simulink model "FCS"  (R2019a)
settings: Solver=VariableStepAuto  StartTime=0.0  StopTime=10.0  RelTol=1e-3
undefined symbols (not defined in the file): argentina, ground, JD_0, Jw, namibia, nut80, r_ecef, t_orbit, v_ecef
libraries: dspmathops x12, vrlib x8, sc_toolbox x7
(part 2 of 2)

== matlab function FCS/Environment/Sun Position Model /MOD to ECEF/MATLAB Function ==
  data: reci input; rteme output; ttt input; ddpsi input; ddeps input; nut80 input
% ----------------------------------------------------------------------------
%
%                           function eci2teme
%
%  this function transforms a vector from the mean equator mean equinox (j2000) 
%    system (eci), to the true equator mean equinox (teme) system.
%
%  author        : david vallado                  719-573-2600   30 oct 2017
%
%  inputs          description                    range / units
%    reci        - position vector eci            km
%    veci        - velocity vector eci            km/s
%    aeci        - acceleration vector eci        km/s2
%    ttt         - julian centuries of tt         centuries
%    ddpsi       - delta psi correction to gcrf   rad
%    ddeps       - delta eps correction to gcrf   rad
%
%  outputs       :
%    rteme       - position vector of date
%                    true equator, mean equinox   km
%    vteme       - velocity vector of date
%                    true equator, mean equinox   km/s
%    ateme       - acceleration vector of date
%                    true equator, mean equinox   km/s2
%
%  locals        :
%    prec        - matrix for eci - mod
%    nutteme     - matrix for mod - teme - an approximation for nutation
%    eqe         - rotation for equation of equinoxes (geometric terms only)
%    tm          - combined matrix for teme2eci
%
%  coupling      :
%   precess      - rotation for precession        eci - mod
%   nutation     - rotation for nutation          eci - tod
%
%  references    :
%    vallado       2013, 231-233
%
% [reci, veci, aeci] = teme2eci  ( rteme, vteme, ateme, ttt, ddpsi, ddeps);
% ----------------------------------------------------------------------------

function rteme  = eci2teme  ( reci, ttt, ddpsi, ddeps, nut80)

        [prec,psia, wa, ea, xa] = precess ( ttt);

        [deltapsi, trueeps, meaneps, omega, nut] = nutation  (ttt, ddpsi, ddeps, nut80 );
        
        % ------------------------ find eqeg ----------------------
        % rotate teme through just geometric terms 
        eqeg = deltapsi* cos(meaneps);

        eqeg = rem (eqeg, 2.0*pi);
        eqe = zeros(3,3);
        eqe(1,1) =  cos(eqeg);
        eqe(1,2) =  sin(eqeg);
        eqe(1,3) =  0.0;
        eqe(2,1) = -sin(eqeg);
        eqe(2,2) =  cos(eqeg);
        eqe(2,3) =  0.0;
        eqe(3,1) =  0.0;
        eqe(3,2) =  0.0;
        eqe(3,3) =  1.0;

        tm = eqe * nut' * prec';
        
        rteme = tm * reci;
 
        


%�
% ----------------------------------------------------------------------------
%
%                           function precess
%
%  this function calulates the transformation matrix that accounts for the effects
%    of precession. both the 1980 and 2000 theories are handled. note that the 
%    required parameters differ a little. 
%
%  author        : david vallado                  719-573-2600   25 jun 2002
%
%  revisions
%    vallado     - consolidate with iau 2000                     14 feb 2005
%
%  inputs          description                    range / units
%    ttt         - julian centuries of tt
%    opt         - method option                  '01', '02', '96', '80'
%
%  outputs       :
%    prec        - transformation matrix for mod - j2000 (80 only)
%    psia        - cannonical precession angle    rad    (00 only)
%    wa          - cannonical precession angle    rad    (00 only)
%    ea          - cannonical precession angle    rad    (00 only)
%    xa          - cannonical precession angle    rad    (00 only)
%
%  locals        :
%    ttt2        - ttt squared
%    ttt3        - ttt cubed
%    zeta        - precession angle               rad
%    z           - precession angle               rad
%    theta       - precession angle               rad
%    oblo        - obliquity value at j2000 epoch "%
%
%  coupling      :
%    none        -
%
%  references    :
%    vallado       2004, 214-216, 219-221
%
% [prec,psia,wa,ea,xa] = precess ( ttt, opt );
% ----------------------------------------------------------------------------

function [prec,psia,wa,ea,xa] = precess ( ttt );

       % sethelp;
        
        % " to rad
        convrt = pi / (180.0*3600.0);
        ttt2= ttt * ttt;
        ttt3= ttt2 * ttt;

        % ------------------- fk4 b1950 precession angles --------------------
%         if (opt == '50')
% 
%             % ---- Seidelmann pg 107             
%             % for these calls, ttt will come in with the current jd
% %            t1= 0.0; %(ttt - 2433282.42345905)/365242.198782;  % set start as B1850, 0.0 to simplify
% %            t2= (ttt - 2396758.203)/365242.198782;  % uses B1850
% %            ttt = t2 - t1;
% %            ttt2 = ttt * ttt;
% %            ttt3 = ttt * ttt2;
% %            fprintf(1,'50prec %15.9f  \n',ttt);
%             % exp supp 61 pg 38
% %            psia = 50.3708 + 0.0050 * ttt;
% %            wa = 0.0;
% %            ea = 0.0;
% %            xa = 0.1247 - 0.0188 * ttt;
% %            zeta =  (23035.545 + 139.720*t1 + 0.060 *t1*t1)*ttt + (30.240-0.270*t1)*ttt2 + 17.995*ttt3; % "
% %            theta=  (20051.12 - 85.29*t1 - 0.37 *t1*t1)*ttt + (-42.65-0.37*t1)*ttt2 - 41.80*ttt3;
% %            z    =  (23035.545 + 139.720*t1 + 0.060 *t1*t1)*ttt + (109.480+0.390*t1)*ttt2 + 18.325*ttt3;
% 
%             % ---- Newcomb Exp Supp 61 approach, but see GTDS pg 3-17
%             % Exp Supp 61 says use 1900? but gtds says use 1950. 
%             % for these calls, ttt will come in with the current jd
%             t1= 0.0; %(ttt - 2415020.31352)/36524.2198782;  % set start as B1900, 0.0 to simplify
% %            t2= (ttt - 2415020.31352)/36525;  % uses B1900   
%             t2= (ttt - 2433282.42345905)/36525;  % uses B1950  
% %            ttt = t2 - t1;
% %            ttt2 = ttt * ttt;
% %            ttt3 = ttt * ttt2;
%             % exp supp 61 pg 38
%             psia = 50.3708 + 0.0050 * ttt;
%             wa = 0.0; % not sure which one is which...
%             ea = 84428.26 -   46.845*ttt - 0.00059*ttt2 + 0.00181*ttt3;
%             xa = 0.1247 - 0.0188 * ttt;
%            fprintf(1,'50prec %15.9f  \n',ttt);
%            % seems like Exp supp 61 is ok with 1900 as epoch, and Seidlemann is ok with listed measr,  
% %            zeta =  (2304.25 + 1.396*t1)*ttt + 0.302*ttt2 + 0.018*ttt3; % "
% %            theta=  (2004.682 - 0.853*t1)*ttt -0.426*ttt2 - 0.042*ttt3;
% %            z    =  (2304.25 + 1.396*t1)*ttt + 1.093*ttt2 + 0.018*ttt3;
%             % GTDS pg 3-17 using days from 1950 - avoids long rpecession
%             % constants...
%             zeta =  2304.9969*ttt + 0.302*ttt2 + 0.01808*ttt3; % "
%             theta=  2004.2980*ttt -0.425936*ttt2 - 0.0416*ttt3;
%             z    =  2304.9969*ttt + 1.092999*ttt2 + 0.0192*ttt3;
%             
% 
%             % tp-008 36-45
%             % ttt is tropical centruies from 1950 36524.22 days
%             prec = zeros(3,3);
%             prec(1,1) =  1.0 - 2.9696e-4 * ttt2 - 1.3e-7 * ttt3;
%             prec(1,2) =  2.234941e-2 * ttt + 6.76e-6 * ttt2 - 2.21e-6 * ttt3;
%             prec(1,3) =  9.7169e-3 * ttt - 2.07e-6 * ttt2 - 9.6e-7 * ttt3;
%             prec(2,1) =  -prec(1,2);
%             prec(2,2) =  1.0 - 2.4975e-4 * ttt2 - 1.5e-7 * ttt3;
%             prec(2,3) =  - 1.0858e-4 * ttt2;
%             prec(3,1) =  -prec(1,3);
%             prec(3,2) =  prec(2,3);
%             prec(3,3) =  1.0 - 4.721e-5 * ttt2;
%  
%             
%            % pass these back out for testing
%            psia = zeta;
%            wa = theta;
%            ea = z;
%         % ------------------- iau 76 precession angles --------------------
%         else
%           if (opt == '80')
%     fprintf(1,'80prec %15.9f  \n',ttt);
            psia =             5038.7784*ttt - 1.07259*ttt2 - 0.001147*ttt3; % "
            wa   = 84381.448                 + 0.05127*ttt2 - 0.007726*ttt3;
            ea   = 84381.448 -   46.8150*ttt - 0.00059*ttt2 + 0.001813*ttt3;
            xa   =               10.5526*ttt - 2.38064*ttt2 - 0.001125*ttt3;
            zeta =             2306.2181*ttt + 0.30188*ttt2 + 0.017998*ttt3; % "
            theta=             2004.3109*ttt - 0.42665*ttt2 - 0.041833*ttt3;
            z    =             2306.2181*ttt + 1.09468*ttt2 + 0.018203*ttt3;
          % ------------------ iau 03 precession angles -------------------
%           else
%             oblo =  84381.406; % "
%             psia =  (((( -0.0000000951 * ttt + 0.000132851 ) * ttt - 0.00114045 ) * ttt - 1.0790069 ) * ttt + 5038.481507 ) * ttt; % "
%             wa   =  ((((  0.0000003337 * ttt - 0.000000467 ) * ttt - 0.00772503 ) * ttt + 0.0512623 ) * ttt -    0.025754 ) * ttt + oblo;
%             ea   =  (((( -0.0000000434 * ttt - 0.000000576 ) * ttt + 0.00200340 ) * ttt - 0.0001831 ) * ttt -   46.836769 ) * ttt + oblo;
%             xa   =  (((( - 0.0000000560 * ttt + 0.000170663 ) * ttt - 0.00121197 ) * ttt - 2.3814292 ) * ttt +   10.556403 ) * ttt;
% 
%             zeta =  (((( - 0.0000003173 * ttt - 0.000005971 ) * ttt + 0.01801828 ) * ttt + 0.2988499 ) * ttt + 2306.083227 ) * ttt + 2.650545; % "
%             theta=  (((( - 0.0000001274 * ttt - 0.000007089 ) * ttt - 0.04182264 ) * ttt - 0.4294934 ) * ttt + 2004.191903 ) * ttt;
%             z    =  ((((   0.0000002904 * ttt - 0.000028596 ) * ttt + 0.01826837 ) * ttt + 1.0927348 ) * ttt + 2306.077181 ) * ttt - 2.650545;
%           end;
%         end;
        
        % convert units to rad
        psia = psia  * convrt; % rad
        wa   = wa    * convrt;
        ea   = ea    * convrt;
        xa   = xa    * convrt;
        zeta = zeta  * convrt; 
        theta= theta * convrt;
        z    = z     * convrt;
%iauhelp='y';         
%fprintf(1,'pr %11.7f  %11.7f  %11.7fdeg \n',zeta*180/pi,theta*180/pi,z*180/pi );
%         if (iauhelp == 'y')
%             fprintf(1,'pr %11.7f  %11.7f  %11.7f %11.7fdeg \n',psia*180/pi,wa*180/pi,ea*180/pi,xa*180/pi );
%             fprintf(1,'pr %11.7f  %11.7f  %11.7fdeg \n',zeta*180/pi,theta*180/pi,z*180/pi );
%         end;
% 
%         if (strcmp(opt,'80')==1) % || (strcmp(opt,'50') == 1)
            coszeta  = cos(zeta);
            sinzeta  = sin(zeta);
            costheta = cos(theta);
            sintheta = sin(theta);
            cosz     = cos(z);
            sinz     = sin(z);

            % ----------------- form matrix  mod to j2000 -----------------
            prec = zeros(3,3);
            prec(1,1) =  coszeta * costheta * cosz - sinzeta * sinz;
            prec(1,2) =  coszeta * costheta * sinz + sinzeta * cosz;
            prec(1,3) =  coszeta * sintheta;
            prec(2,1) = -sinzeta * costheta * cosz - coszeta * sinz;
            prec(2,2) = -sinzeta * costheta * sinz + coszeta * cosz;
            prec(2,3) = -sinzeta * sintheta;
            prec(3,1) = -sintheta * cosz;
            prec(3,2) = -sintheta * sinz;
            prec(3,3) =  costheta;

            % ----------------- do rotations instead ----------------------
            % p1 = rot3mat( z );
            % p2 = rot2mat( -theta );
            % p3 = rot3mat( zeta );
            % prec = p3*p2*p1;
%         elseif (strcmp(opt,'50') ~= 1)
%             oblo = oblo * convrt; % " to rad
%             a4  = rot3mat(-xa);
%             a5  = rot1mat(wa);
%             a6  = rot3mat(psia);
%             a7  = rot1mat(-oblo);
%             prec = a7*a6*a5*a4;
%            % prec = zeros(3);
%         end;



% ----------------------------------------------------------------------------
%
%                           function nutation
%
%  this function calulates the transformation matrix that accounts for the
%    effects of nutation.
%
%  author        : david vallado                  719-573-2600   27 jun 2002
%
%  revisions
%    vallado     - consolidate with iau 2000                     14 feb 2005
%
%  inputs          description                    range / units
%    ttt         - julian centuries of tt
%    ddpsi       - delta psi correction to gcrf   rad
%    ddeps       - delta eps correction to gcrf   rad
%
%  outputs       :
%    deltapsi    - nutation angle                 rad
%    trueeps     - true obliquity of the ecliptic rad
%    meaneps     - mean obliquity of the ecliptic rad
%    omega       -                                rad
%    nut         - transformation matrix for tod - mod
%
%  locals        :
%    iar80       - integers for fk5 1980
%    rar80       - reals for fk5 1980
%    ttt2        - ttt squared
%    ttt3        - ttt cubed
%    l           -                                rad
%    ll          -                                rad
%    f           -                                rad
%    d           -                                rad
%    deltaeps    - change in obliquity            rad
%
%  coupling      :
%    fundarg     - find fundamental arguments
%
%  references    :
%    vallado       2013, 224-226
%
% [deltapsi, trueeps, meaneps, omega,nut] = nutation  (ttt, ddpsi, ddeps );
% ----------------------------------------------------------------------------

function [deltapsi, trueeps, meaneps, omega,nut] = nutation  (ttt, ddpsi, ddeps , nut80);

        deg2rad = pi/180.0;

        [iar80,rar80] =  iau80in(nut80);  % coeff in deg

        % ---- determine coefficients for iau 1980 nutation theory ----
        ttt2= ttt*ttt;
        ttt3= ttt2*ttt;

        meaneps = -46.8150 *ttt - 0.00059 *ttt2 + 0.001813 *ttt3 + 84381.448;
        meaneps = rem( meaneps/3600.0, 360.0 );
        meaneps = meaneps * deg2rad;

        [ l, l1, f, d, omega, ...
          lonmer, lonven, lonear, lonmar, lonjup, lonsat, lonurn, lonnep, precrate ...
        ] = fundarg( ttt, '80' );
%fprintf(1,'nut del arg %11.7f  %11.7f  %11.7f  %11.7f  %11.7f  \n',l*180/pi,l1*180/pi,f*180/pi,d*180/pi,omega*180/pi );

        deltapsi= 0.0;
        deltaeps= 0.0;
        for i= 106:-1: 1
            tempval= iar80(i,1)*l + iar80(i,2)*l1 + iar80(i,3)*f + ...
                     iar80(i,4)*d + iar80(i,5)*omega;
            deltapsi= deltapsi + (rar80(i,1)+rar80(i,2)*ttt) * sin( tempval );
            deltaeps= deltaeps + (rar80(i,3)+rar80(i,4)*ttt) * cos( tempval );
        end

        % --------------- find nutation parameters --------------------
        deltapsi = rem( deltapsi + ddpsi, 2.0 * pi );
        deltaeps = rem( deltaeps + ddeps, 2.0 * pi );
        trueeps  = meaneps + deltaeps;

%fprintf(1,'meaneps %11.7f dp  %11.7f de  %11.7f te  %11.7f  ttt  %11.7f \n',meaneps*180/pi,deltapsi*180/pi,deltaeps*180/pi,trueeps*180/pi, ttt );

        cospsi  = cos(deltapsi);
        sinpsi  = sin(deltapsi);
        coseps  = cos(meaneps);
        sineps  = sin(meaneps);
        costrueeps = cos(trueeps);
        sintrueeps = sin(trueeps);
        
        nut = zeros(3,3);
        nut(1,1) =  cospsi;
        nut(1,2) =  costrueeps * sinpsi;
        nut(1,3) =  sintrueeps * sinpsi;
        nut(2,1) = -coseps * sinpsi;
        nut(2,2) =  costrueeps * coseps * cospsi + sintrueeps * sineps;
        nut(2,3) =  sintrueeps * coseps * cospsi - sineps * costrueeps;
        nut(3,1) = -sineps * sinpsi;
        nut(3,2) =  costrueeps * sineps * cospsi - sintrueeps * coseps;
        nut(3,3) =  sintrueeps * sineps * cospsi + costrueeps * coseps;

      %   n1 = rot1mat( trueeps );
      %   n2 = rot3mat( deltapsi );
      %   n3 = rot1mat( -meaneps );
      %   nut = n3*n2*n1

%�
% ----------------------------------------------------------------------------
%
%                           function fundarg
%
%  this function calulates the delauany variables and planetary values for
%  several theories.
%
%  author        : david vallado                  719-573-2600   16 jul 2004
%
%  revisions
%    vallado     - consolidate with iau 2000                     14 feb 2005
%
%  inputs          description                    range / units
%    ttt         - julian centuries of tt
%    opt         - method option                  '10', '02', '96', '80'
%
%  outputs       :
%    l           - delaunay element               rad
%    ll          - delaunay element               rad
%    f           - delaunay element               rad
%    d           - delaunay element               rad
%    omega       - delaunay element               rad
%    planetary longitudes                         rad
%
%  locals        :
%    ttt2,ttt3,  - powers of ttt
%
%  coupling      :
%    none        -
%
%  references    :
%    vallado       2004, 212-214
%
% [ l, l1, f, d, omega, ...
%   lonmer, lonven, lonear, lonmar, lonjup, lonsat, lonurn, lonnep, precrate ...
% ] = fundarg( ttt, opt );
% ----------------------------------------------------------------------------

function [ l, l1, f, d, omega, ...
           lonmer, lonven, lonear, lonmar, lonjup, lonsat, lonurn, lonnep, precrate ...
         ] = fundarg( ttt, opt )

        %sethelp;

        deg2rad = pi/180.0;

        % ---- determine coefficients for iau 2000 nutation theory ----
        ttt2 = ttt*ttt;
        ttt3 = ttt2*ttt;
        ttt4 = ttt2*ttt2;

        % ---- iau 2010 theory
        if opt == '10'
            % ------ form the delaunay fundamental arguments in deg
            l    =  134.96340251  + ( 1717915923.2178 *ttt + ...
                     31.8792 *ttt2 + 0.051635 *ttt3 - 0.00024470 *ttt4 ) / 3600.0;
            l1   =  357.52910918  + (  129596581.0481 *ttt - ...
                      0.5532 *ttt2 - 0.000136 *ttt3 - 0.00001149*ttt4 )  / 3600.0;
            f    =   93.27209062  + ( 1739527262.8478 *ttt - ...
                     12.7512 *ttt2 + 0.001037 *ttt3 + 0.00000417*ttt4 )  / 3600.0;
            d    =  297.85019547  + ( 1602961601.2090 *ttt - ...
                      6.3706 *ttt2 + 0.006593 *ttt3 - 0.00003169*ttt4 )  / 3600.0;
            omega=  125.04455501  + (   -6962890.5431 *ttt + ...
                      7.4722 *ttt2 + 0.007702 *ttt3 - 0.00005939*ttt4 )  / 3600.0;

            % ------ form the planetary arguments in deg
            lonmer  = 252.250905494  + 149472.6746358  *ttt;
            lonven  = 181.979800853  +  58517.8156748  *ttt;
            lonear  = 100.466448494  +  35999.3728521  *ttt;
            lonmar  = 355.433274605  +  19140.299314   *ttt;
            lonjup  =  34.351483900  +   3034.90567464 *ttt;
            lonsat  =  50.0774713998 +   1222.11379404 *ttt;
            lonurn  = 314.055005137  +    428.466998313*ttt;
            lonnep  = 304.348665499  +    218.486200208*ttt;
            precrate=   1.39697137214*ttt + 0.0003086*ttt2;
         end;

        % ---- iau 2000b theory
        if opt == '02'
            % ------ form the delaunay fundamental arguments in deg
            l    =  134.96340251  + ( 1717915923.2178 *ttt ) / 3600.0;
            l1   =  357.52910918  + (  129596581.0481 *ttt ) / 3600.0;
            f    =   93.27209062  + ( 1739527262.8478 *ttt ) / 3600.0;
            d    =  297.85019547  + ( 1602961601.2090 *ttt ) / 3600.0;
            omega=  125.04455501  + (   -6962890.5431 *ttt ) / 3600.0;

            % ------ form the planetary arguments in deg
            lonmer  = 0.0;
            lonven  = 0.0;
            lonear  = 0.0;
            lonmar  = 0.0;
            lonjup  = 0.0;
            lonsat  = 0.0;
            lonurn  = 0.0;
            lonnep  = 0.0;
            precrate= 0.0;
         end;   

        % ---- iau 1996 theory
        if opt == '96'
            l    =  134.96340251  + ( 1717915923.2178 *ttt + ...
                     31.8792 *ttt2 + 0.051635 *ttt3 - 0.00024470 *ttt4 ) / 3600.0;
            l1   =  357.52910918  + (  129596581.0481 *ttt - ...
                      0.5532 *ttt2 - 0.000136 *ttt3 - 0.00001149*ttt4 )  / 3600.0;
            f    =   93.27209062  + ( 1739527262.8478 *ttt - ...
                     12.7512 *ttt2 + 0.001037 *ttt3 + 0.00000417*ttt4 )  / 3600.0;
            d    =  297.85019547  + ( 1602961601.2090 *ttt - ...
                      6.3706 *ttt2 + 0.006593 *ttt3 - 0.00003169*ttt4 )  / 3600.0;
            omega=  125.04455501  + (   -6962890.2665 *ttt + ...
                      7.4722 *ttt2 + 0.007702 *ttt3 - 0.00005939*ttt4 )  / 3600.0;
            % ------ form the planetary arguments in deg
            lonmer  = 0.0;
            lonven  = 181.979800853  +  58517.8156748  *ttt;   % deg
            lonear  = 100.466448494  +  35999.3728521  *ttt;
            lonmar  = 355.433274605  +  19140.299314   *ttt;
            lonjup  =  34.351483900  +   3034.90567464 *ttt;
            lonsat  =  50.0774713998 +   1222.11379404 *ttt;
            lonurn  = 0.0;
            lonnep  = 0.0;
            precrate=   1.39697137214*ttt + 0.0003086*ttt2;
         end;   

         % ---- iau 1980 theory
        if opt == '80'
            l = ((((0.064) * ttt + 31.310) * ttt + 1717915922.6330) * ttt) / 3600.0 + 134.96298139;
    		l1 = ((((-0.012) * ttt - 0.577) * ttt + 129596581.2240) * ttt) / 3600.0 + 357.52772333;
    		f = ((((0.011) * ttt - 13.257) * ttt + 1739527263.1370) * ttt) / 3600.0 + 93.27191028;
	    	d = ((((0.019) * ttt - 6.891) * ttt + 1602961601.3280) * ttt) / 3600.0 + 297.85036306;
    		omega = ((((0.008) * ttt + 7.455) * ttt - 6962890.5390) * ttt) / 3600.0 + 125.04452222;
                  
            % ------ form the planetary arguments in deg
            lonmer  = 252.3 + 149472.0 *ttt;
            lonven  = 179.9 +  58517.8 *ttt;   % deg
            lonear  =  98.4 +  35999.4 *ttt;
            lonmar  = 353.3 +  19140.3 *ttt;
            lonjup  =  32.3 +   3034.9 *ttt;
            lonsat  =  48.0 +   1222.1 *ttt;
            lonurn  =   0.0;
            lonnep  =   0.0;
            precrate=   0.0;
         end;   

        % ---- convert units to rad
        l    = rem( l,360.0  )     * deg2rad; % rad
        l1   = rem( l1,360.0  )    * deg2rad;
        f    = rem( f,360.0  )     * deg2rad;
        d    = rem( d,360.0  )     * deg2rad;
        omega= rem( omega,360.0  ) * deg2rad;

        lonmer= rem( lonmer,360.0 ) * deg2rad;  % rad
        lonven= rem( lonven,360.0 ) * deg2rad;
        lonear= rem( lonear,360.0 ) * deg2rad;
        lonmar= rem( lonmar,360.0 ) * deg2rad;
        lonjup= rem( lonjup,360.0 ) * deg2rad;
        lonsat= rem( lonsat,360.0 ) * deg2rad;
        lonurn= rem( lonurn,360.0 ) * deg2rad;
        lonnep= rem( lonnep,360.0 ) * deg2rad;
        precrate= rem( precrate,360.0 ) * deg2rad;
%iauhelp='y';
%         if iauhelp == 'y'
%             fprintf(1,'fa %11.7f  %11.7f  %11.7f  %11.7f  %11.7f deg \n',l*180/pi,l1*180/pi,f*180/pi,d*180/pi,omega*180/pi );
%             fprintf(1,'fa %11.7f  %11.7f  %11.7f  %11.7f deg \n',lonmer*180/pi,lonven*180/pi,lonear*180/pi,lonmar*180/pi );
%             fprintf(1,'fa %11.7f  %11.7f  %11.7f  %11.7f deg \n',lonjup*180/pi,lonsat*180/pi,lonurn*180/pi,lonnep*180/pi );
%             fprintf(1,'fa %11.7f  \n',precrate*180/pi );
%           end;

function [iar80,rar80] = iau80in(nut80);

       % ------------------------  implementation   -------------------
       % 0.0001" to rad
       convrt= 0.0001 * pi / (180*3600.0);

       %load nut80.dat;

       iar80 = nut80(:,1:5);
       rar80 = nut80(:,6:9);

       for i=1:106
           for j=1:4
               rar80(i,j)= rar80(i,j) * convrt;
           end
       end

== matlab function FCS/Environment/Sun Position Model /MOD to ECEF/MOD to ECI ==
  data: rmod input; reci output; ttt input
% ----------------------------------------------------------------------------
%
%                           function mod2eci
%
%  this function transforms a vector from the mean equator mean equinox of
%    date (mod) to the mean equator mean equinox (j2000) frame.
%
%  author        : david vallado                  719-573-2600   25 jun 2002
%
%  revisions
%    vallado     - consolidate with iau 2000                     14 feb 2005
%
%  inputs          description                    range / units
%    rmod        - position vector of date
%                    mean equator, mean equinox   km
%    vmod        - velocity vector of date
%                    mean equator, mean equinox   km/s
%    amod        - acceleration vector of date
%                    mean equator, mean equinox   km/s2
%    ttt         - julian centuries of tt         centuries
%
%  outputs       :
%    reci        - position vector eci            km
%    veci        - velocity vector eci            km/s
%    aeci        - acceleration vector eci        km/s2
%
%  locals        :
%    none.
%
%  coupling      :
%   precess      - rotation for precession        mod - eci
%
%  references    :
%    vallado       2001, 219-220, eq 3-68
%
% [reci,veci,aeci] = mod2eci  ( rmod,vmod,amod,ttt );
% ----------------------------------------------------------------------------

function reci  = mod2eci  ( rmod,ttt )
        
        
        [prec,psia,wa,ea,xa] = precess1 ( ttt);

        reci = prec*rmod;
        
        
        
        
        % ----------------------------------------------------------------------------
%
%                           function precess
%
%  this function calulates the transformation matrix that accounts for the effects
%    of precession. both the 1980 and 2000 theories are handled. note that the 
%    required parameters differ a little. 
%
%  author        : david vallado                  719-573-2600   25 jun 2002
%
%  revisions
%    vallado     - consolidate with iau 2000                     14 feb 2005
%
%  inputs          description                    range / units
%    ttt         - julian centuries of tt
%    opt         - method option                  '01', '02', '96', '80'
%
%  outputs       :
%    prec        - transformation matrix for mod - j2000 (80 only)
%    psia        - cannonical precession angle    rad    (00 only)
%    wa          - cannonical precession angle    rad    (00 only)
%    ea          - cannonical precession angle    rad    (00 only)
%    xa          - cannonical precession angle    rad    (00 only)
%
%  locals        :
%    ttt2        - ttt squared
%    ttt3        - ttt cubed
%    zeta        - precession angle               rad
%    z           - precession angle               rad
%    theta       - precession angle               rad
%    oblo        - obliquity value at j2000 epoch "%
%
%  coupling      :
%    none        -
%
%  references    :
%    vallado       2004, 214-216, 219-221
%
% [prec,psia,wa,ea,xa] = precess ( ttt, opt );
% ----------------------------------------------------------------------------

function [prec,psia,wa,ea,xa] = precess1 ( ttt );

       % sethelp;
        
        % " to rad
        convrt = pi / (180.0*3600.0);
        ttt2= ttt * ttt;
        ttt3= ttt2 * ttt;

        % ------------------- fk4 b1950 precession angles --------------------
%         if (opt == '50')
% 
%             % ---- Seidelmann pg 107             
%             % for these calls, ttt will come in with the current jd
% %            t1= 0.0; %(ttt - 2433282.42345905)/365242.198782;  % set start as B1850, 0.0 to simplify
% %            t2= (ttt - 2396758.203)/365242.198782;  % uses B1850
% %            ttt = t2 - t1;
% %            ttt2 = ttt * ttt;
% %            ttt3 = ttt * ttt2;
% %            fprintf(1,'50prec %15.9f  \n',ttt);
%             % exp supp 61 pg 38
% %            psia = 50.3708 + 0.0050 * ttt;
% %            wa = 0.0;
% %            ea = 0.0;
% %            xa = 0.1247 - 0.0188 * ttt;
% %            zeta =  (23035.545 + 139.720*t1 + 0.060 *t1*t1)*ttt + (30.240-0.270*t1)*ttt2 + 17.995*ttt3; % "
% %            theta=  (20051.12 - 85.29*t1 - 0.37 *t1*t1)*ttt + (-42.65-0.37*t1)*ttt2 - 41.80*ttt3;
% %            z    =  (23035.545 + 139.720*t1 + 0.060 *t1*t1)*ttt + (109.480+0.390*t1)*ttt2 + 18.325*ttt3;
% 
%             % ---- Newcomb Exp Supp 61 approach, but see GTDS pg 3-17
%             % Exp Supp 61 says use 1900? but gtds says use 1950. 
%             % for these calls, ttt will come in with the current jd
%             t1= 0.0; %(ttt - 2415020.31352)/36524.2198782;  % set start as B1900, 0.0 to simplify
% %            t2= (ttt - 2415020.31352)/36525;  % uses B1900   
%             t2= (ttt - 2433282.42345905)/36525;  % uses B1950  
% %            ttt = t2 - t1;
% %            ttt2 = ttt * ttt;
% %            ttt3 = ttt * ttt2;
%             % exp supp 61 pg 38
%             psia = 50.3708 + 0.0050 * ttt;
%             wa = 0.0; % not sure which one is which...
%             ea = 84428.26 -   46.845*ttt - 0.00059*ttt2 + 0.00181*ttt3;
%             xa = 0.1247 - 0.0188 * ttt;
%            fprintf(1,'50prec %15.9f  \n',ttt);
%            % seems like Exp supp 61 is ok with 1900 as epoch, and Seidlemann is ok with listed measr,  
% %            zeta =  (2304.25 + 1.396*t1)*ttt + 0.302*ttt2 + 0.018*ttt3; % "
% %            theta=  (2004.682 - 0.853*t1)*ttt -0.426*ttt2 - 0.042*ttt3;
% %            z    =  (2304.25 + 1.396*t1)*ttt + 1.093*ttt2 + 0.018*ttt3;
%             % GTDS pg 3-17 using days from 1950 - avoids long rpecession
%             % constants...
%             zeta =  2304.9969*ttt + 0.302*ttt2 + 0.01808*ttt3; % "
%             theta=  2004.2980*ttt -0.425936*ttt2 - 0.0416*ttt3;
%             z    =  2304.9969*ttt + 1.092999*ttt2 + 0.0192*ttt3;
%             
% 
%             % tp-008 36-45
%             % ttt is tropical centruies from 1950 36524.22 days
%             prec = zeros(3,3);
%             prec(1,1) =  1.0 - 2.9696e-4 * ttt2 - 1.3e-7 * ttt3;
%             prec(1,2) =  2.234941e-2 * ttt + 6.76e-6 * ttt2 - 2.21e-6 * ttt3;
%             prec(1,3) =  9.7169e-3 * ttt - 2.07e-6 * ttt2 - 9.6e-7 * ttt3;
%             prec(2,1) =  -prec(1,2);
%             prec(2,2) =  1.0 - 2.4975e-4 * ttt2 - 1.5e-7 * ttt3;
%             prec(2,3) =  - 1.0858e-4 * ttt2;
%             prec(3,1) =  -prec(1,3);
%             prec(3,2) =  prec(2,3);
%             prec(3,3) =  1.0 - 4.721e-5 * ttt2;
%  
%             
%            % pass these back out for testing
%            psia = zeta;
%            wa = theta;
%            ea = z;
%         % ------------------- iau 76 precession angles --------------------
%         else
%           if (opt == '80')
%     fprintf(1,'80prec %15.9f  \n',ttt);
            psia =             5038.7784*ttt - 1.07259*ttt2 - 0.001147*ttt3; % "
            wa   = 84381.448                 + 0.05127*ttt2 - 0.007726*ttt3;
            ea   = 84381.448 -   46.8150*ttt - 0.00059*ttt2 + 0.001813*ttt3;
            xa   =               10.5526*ttt - 2.38064*ttt2 - 0.001125*ttt3;
            zeta =             2306.2181*ttt + 0.30188*ttt2 + 0.017998*ttt3; % "
            theta=             2004.3109*ttt - 0.42665*ttt2 - 0.041833*ttt3;
            z    =             2306.2181*ttt + 1.09468*ttt2 + 0.018203*ttt3;
          % ------------------ iau 03 precession angles -------------------
%           else
%             oblo =  84381.406; % "
%             psia =  (((( -0.0000000951 * ttt + 0.000132851 ) * ttt - 0.00114045 ) * ttt - 1.0790069 ) * ttt + 5038.481507 ) * ttt; % "
%             wa   =  ((((  0.0000003337 * ttt - 0.000000467 ) * ttt - 0.00772503 ) * ttt + 0.0512623 ) * ttt -    0.025754 ) * ttt + oblo;
%             ea   =  (((( -0.0000000434 * ttt - 0.000000576 ) * ttt + 0.00200340 ) * ttt - 0.0001831 ) * ttt -   46.836769 ) * ttt + oblo;
%             xa   =  (((( - 0.0000000560 * ttt + 0.000170663 ) * ttt - 0.00121197 ) * ttt - 2.3814292 ) * ttt +   10.556403 ) * ttt;
% 
%             zeta =  (((( - 0.0000003173 * ttt - 0.000005971 ) * ttt + 0.01801828 ) * ttt + 0.2988499 ) * ttt + 2306.083227 ) * ttt + 2.650545; % "
%             theta=  (((( - 0.0000001274 * ttt - 0.000007089 ) * ttt - 0.04182264 ) * ttt - 0.4294934 ) * ttt + 2004.191903 ) * ttt;
%             z    =  ((((   0.0000002904 * ttt - 0.000028596 ) * ttt + 0.01826837 ) * ttt + 1.0927348 ) * ttt + 2306.077181 ) * ttt - 2.650545;
%           end;
%         end;
        
        % convert units to rad
        psia = psia  * convrt; % rad
        wa   = wa    * convrt;
        ea   = ea    * convrt;
        xa   = xa    * convrt;
        zeta = zeta  * convrt; 
        theta= theta * convrt;
        z    = z     * convrt;
%iauhelp='y';         
%fprintf(1,'pr %11.7f  %11.7f  %11.7fdeg \n',zeta*180/pi,theta*180/pi,z*180/pi );
%         if (iauhelp == 'y')
%             fprintf(1,'pr %11.7f  %11.7f  %11.7f %11.7fdeg \n',psia*180/pi,wa*180/pi,ea*180/pi,xa*180/pi );
%             fprintf(1,'pr %11.7f  %11.7f  %11.7fdeg \n',zeta*180/pi,theta*180/pi,z*180/pi );
%         end;
% 
%         if (strcmp(opt,'80')==1) % || (strcmp(opt,'50') == 1)
            coszeta  = cos(zeta);
            sinzeta  = sin(zeta);
            costheta = cos(theta);
            sintheta = sin(theta);
            cosz     = cos(z);
            sinz     = sin(z);

            % ----------------- form matrix  mod to j2000 -----------------
            prec = zeros(3,3);
            prec(1,1) =  coszeta * costheta * cosz - sinzeta * sinz;
            prec(1,2) =  coszeta * costheta * sinz + sinzeta * cosz;
            prec(1,3) =  coszeta * sintheta;
            prec(2,1) = -sinzeta * costheta * cosz - coszeta * sinz;
            prec(2,2) = -sinzeta * costheta * sinz + coszeta * cosz;
            prec(2,3) = -sinzeta * sintheta;
            prec(3,1) = -sintheta * cosz;
            prec(3,2) = -sintheta * sinz;
            prec(3,3) =  costheta;

== matlab function FCS/Environment/Sun Position Model /Sun Position Vector ==
  data: jd input; rsun output
% ------------------------------------------------------------------------------
%
%                           function sun
%
%  this function calculates the geocentric equatorial position vector
%    the sun given the julian date.  this is the low precision formula and
%    is valid for years from 1950 to 2050.  accuaracy of apparent coordinates
%    is 0.01  degrees.  notice many of the calculations are performed in
%    degrees, and are not changed until later.  this is due to the fact that
%    the almanac uses degrees exclusively in their formulations.
%
%  author        : david vallado                  719-573-2600   27 may 2002
%
%  revisions
%    vallado     - fix mean lon of sun                            7 mat 2004
%
%  inputs          description                    range / units
%    jd          - julian date in UTC             days from 4713 bc
%
%  outputs       :
%    rsun        - ijk position vector of the sun au
%    rtasc       - right ascension                rad
%    decl        - declination                    rad
%
%  locals        :
%    meanlong    - mean longitude
%    meananomaly - mean anomaly
%    eclplong    - ecliptic longitude
%    obliquity   - mean obliquity of the ecliptic
%    tut1        - julian centuries of ut1 from
%                  jan 1, 2000 12h
%    ttdb        - julian centuries of tdb from
%                  jan 1, 2000 12h
%    hr          - hours                          0 .. 24              10
%    min         - minutes                        0 .. 59              15
%    sec         - seconds                        0.0  .. 59.99          30.00
%    temp        - temporary variable
%    deg         - degrees
%
%  coupling      :
%    none.
%
%  references    :
%    vallado       2007, 281, alg 29, ex 5-1
%
% [rsun,rtasc,decl] = sun ( jd );
% ------------------------------------------------------------------------------

function rsun  = sun ( jd )

        twopi      =     2.0*pi;
        deg2rad    =     pi/180.0;
        show = 'n';
        
        % -------------------------  implementation   -----------------
        % -------------------  initialize values   --------------------
        tut1= ( jd - 2451545.0  )/ 36525.0;

        if show == 'y'
            fprintf(1,'tut1 %14.9f \n',tut1);
        end

        meanlong= 280.460  + 36000.77*tut1;
        meanlong= rem( meanlong,360.0  );  %deg

        ttdb= tut1;
        meananomaly= 357.5277233  + 35999.05034 *ttdb;
        meananomaly= rem( meananomaly*deg2rad,twopi );  %rad
        if ( meananomaly < 0.0  )
            meananomaly= twopi + meananomaly;
        end

        eclplong= meanlong + 1.914666471 *sin(meananomaly) ...
                    + 0.019994643 *sin(2.0 *meananomaly); %deg
        eclplong= rem( eclplong,360.0  );  %deg

        obliquity= 23.439291  - 0.0130042 *ttdb;  %deg

        eclplong = eclplong *deg2rad;
        obliquity= obliquity *deg2rad;

        % --------- find magnitude of sun vector, )   components ------
        magr= 1.000140612  - 0.016708617 *cos( meananomaly ) ...
                              - 0.000139589 *cos( 2.0 *meananomaly );    % in au's
        rsun = zeros(3,1);
        rsun(1)= magr*cos( eclplong );
        rsun(2)= magr*cos(obliquity)*sin(eclplong);
        rsun(3)= magr*sin(obliquity)*sin(eclplong);

        if show == 'y'
            fprintf(1,'meanlon %11.6f meanan %11.6f eclplon %11.6f obli %11.6f \n', ...
                    meanlong,meananomaly/deg2rad,eclplong/deg2rad,obliquity/deg2rad);
            fprintf(1,'rs %11.9f %11.9f %11.9f \n',rsun);
            fprintf(1,'magr %14.7f \n',magr);
        end

        rtasc= atan( cos(obliquity)*tan(eclplong) );

        % --- check that rtasc is in the same quadrant as eclplong ----
        if ( eclplong < 0.0  )
            eclplong= eclplong + twopi;    % make sure it's in 0 to 2pi range
        end
        if ( abs( eclplong-rtasc ) > pi*0.5  )
            rtasc= rtasc + 0.5 *pi*round( (eclplong-rtasc)/(0.5 *pi));
        end
        decl = asin( sin(obliquity)*sin(eclplong) );

== matlab function FCS/Environment/Sun Position Model /MOD to ECEF/MATLAB Function1 ==
  data: rteme input; recef output; ttt input; jdut1 input; lod input; xp input; yp input; eqeterms input
% ----------------------------------------------------------------------------
%
%                           function teme2ecef
%
%  this function trsnforms a vector from the true equator mean equniox frame
%    (teme), to an earth fixed (ITRF) frame.  the results take into account
%    the effects of sidereal time, and polar motion.
%
%  author        : david vallado                  719-573-2600   30 oct 2017
%
%  revisions
%
%  inputs          description                    range / units
%    rteme       - position vector teme           km
%    vteme       - velocity vector teme           km/s
%    ateme       - acceleration vector teme (if available, else set to 0)      km/s2
%    ttt         - julian centuries of tt         centuries
%    jdut1       - julian date of ut1             days from 4713 bc
%    lod         - excess length of day           sec
%    xp          - polar motion coefficient       rad
%    yp          - polar motion coefficient       rad
%    eqeterms    - use extra two terms (kinematic) after 1997  0, 2
%
%  outputs       :
%    recef       - position vector earth fixed    km
%    vecef       - velocity vector earth fixed    km/s
%    aecef       - acceleration vector earth fixedkm/s2
%
%  locals        :
%    st          - matrix for pef - tod 
%    pm          - matrix for ecef - pef 
%
%  coupling      :
%   gstime       - greenwich mean sidereal time   rad
%   polarm       - rotation for polar motion      pef - ecef
%
%  references    :
%    vallado       2013, 231-233
%
% [recef, vecef, aecef] = teme2ecef( rteme, vteme, ateme, ttt, jdut1, lod, xp, yp, eqeterms );
% ----------------------------------------------------------------------------

function recef  = teme2ecef( rteme, ttt, jdut1, lod, xp, yp, eqeterms )

        deg2rad = pi/180.0;
        
        % ------------------------ find gmst --------------------------
        gmst= gstime( jdut1 );

        % find omega from nutation theory
        omega=  125.04452222  + (   -6962890.5390 *ttt + ...
                7.455 *ttt*ttt + 0.008 *ttt*ttt*ttt )  / 3600.0;
        omega= rem( omega, 360.0  ) * deg2rad;
        
        % ------------------------ find mean ast ----------------------
        % teme does not include the geometric terms here
        % after 1997, kinematic terms apply
        if (jdut1 > 2450449.5 ) && (eqeterms > 0)
            gmstg = gmst ...
                   + 0.00264*pi /(3600*180)*sin(omega) ...
                   + 0.000063*pi /(3600*180)*sin(2.0 *omega);
        else
            gmstg = gmst;
        end

        gmstg = rem (gmstg, 2.0*pi);
        st = zeros(3,3);
        st(1,1) =  cos(gmstg);
        st(1,2) = -sin(gmstg);
        st(1,3) =  0.0;
        st(2,1) =  sin(gmstg);
        st(2,2) =  cos(gmstg);
        st(2,3) =  0.0;
        st(3,1) =  0.0;
        st(3,2) =  0.0;
        st(3,3) =  1.0;

        [pm] = polarm(xp,yp,ttt,'80');

        rpef  = st'*rteme;
        recef = pm'*rpef;




function [pm] = polarm ( xp, yp, ttt, opt )


        cosxp = cos(xp);
        sinxp = sin(xp);
        cosyp = cos(yp);
        sinyp = sin(yp);

        if (opt == '80')
            pm = zeros(3,3);
            pm(1,1) =  cosxp;
            pm(1,2) =  0.0;
            pm(1,3) = -sinxp;
            pm(2,1) =  sinxp * sinyp;
            pm(2,2) =  cosyp;
            pm(2,3) =  cosxp * sinyp;
            pm(3,1) =  sinxp * cosyp;
            pm(3,2) = -sinyp;
            pm(3,3) =  cosxp * cosyp;

            % a1 = rot2mat(xp);
            % a2 = rot1mat(yp);
            % pm = a2*a1;          
            % Approximate matrix using small angle approximations
            %pm(1,1) =  1.0;
            %pm(2,1) =  0.0;
            %pm(3,1) =  xp;
            %pm(1,2) =  0.0;
            %pm(2,2) =  1.0;
            %pm(3,2) = -yp;
            %pm(1,3) = -xp;
            %pm(2,3) =  yp;
            %pm(3,3) =  1.0;
        else  
            convrt = pi / (3600.0*180.0);
            % approximate sp value in rad
            sp = -47.0e-6 * ttt * convrt;
            cossp = cos(sp);
            sinsp = sin(sp);

            % form the matrix
            pm = zeros(3,3);
            pm(1,1) =  cosxp * cossp;
            pm(1,2) = -cosyp * sinsp + sinyp * sinxp * cossp;
            pm(1,3) = -sinyp * sinsp - cosyp * sinxp * cossp;
            pm(2,1) =  cosxp * sinsp;
            pm(2,2) =  cosyp * cossp + sinyp * sinxp * sinsp;
            pm(2,3) =  sinyp * cossp - cosyp * sinxp * sinsp;
            pm(3,1) =  sinxp;
            pm(3,2) = -sinyp * cosxp;
            pm(3,3) =  cosyp * cosxp;

            % a1 = rot1mat(yp);
            % a2 = rot2mat(xp);
            % a3 = rot3mat(-sp);
            % pm = a3*a2*a1;
        end

== matlab function FCS/Guidance/Reference DCM Computation1 ==
  data: Mode input; DCM_ref output; sun_L input
function DCM_ref = fcn(Mode, sun_L)

switch Mode
    case 1 %Sun
        
        a = atan2(sun_L(3),sun_L(1));
        
        T1 = [0 0 -1;
            0 1 0;
            1 0 0];
        
        T2 = [cos(a) 0 sin(a);
            0 1 0;
            -sin(a) 0 cos(a)];
        
        T3 = [cos(pi/4) sin(pi/4) 0;
            -sin(pi/4) cos(pi/4) 0;
            0 0 1];
        
        DCM_ref = T3*T2*T1;
        
        
    case 2 %Ground
                  
        DCM_ref = [-1 0 0;
                    0 1 0;
                    0 0 -1];
        
    case 3 %Argentina
        
        T1 = [1 0 0;
            0 0 1;
            0 -1 0];
        T3 = [0 1 0;
            -1 0 0;
            0 0 1];
        
        DCM_ref = T1*T3;
        
    case 4 %Namibia
        T1 = [1 0 0;
            0 0 1;
            0 -1 0];
        T3 = [0 1 0;
            -1 0 0;
            0 0 1];
        
        DCM_ref = T1*T3;
        
    otherwise %Nadir
        T1 = [1 0 0;
            0 0 1;
            0 -1 0];
        T3 = [0 1 0;
            -1 0 0;
            0 0 1];
        
        DCM_ref = T1*T3;
        
end

== matlab function FCS/Guidance/Mode Selector ==
  data: N input; G input; A input; P input; Eclipse input; Mode output; Ltot input
function Mode  = Selector(N, G, A,P,Eclipse,Ltot)

persistent Mode_i
if isempty(Mode_i)
    Mode_i = 7;%OFF
end

if Mode_i == 6 && norm(Ltot) > 0.9e-3 %bdot exit criteria
   Mode_i = 6; %Detumbling
elseif max(abs(Ltot)) > 1.7e-3 %saturation
   Mode_i = 6; %Detumbling 
elseif Eclipse == 1 %twilight
   Mode_i = 5; %Nadir Pointing
elseif dot(P,A)/(norm(P)*norm(A)) > 0.96 %In range of Argentina
   Mode_i = 3; %Imaging Argentina
elseif dot(P,N)/(norm(P)*norm(N)) > 0.96 %In range of Namibia
   Mode_i = 4; %Imaging Namibia 
elseif dot(P,G)/(norm(P)*norm(G)) > 0.91 %In range of ground
   Mode_i = 2; %Ground
else %default
   Mode_i = 1; %Sun
end


Mode = Mode_i;

== matlab function FCS/Guidance/Guidance ==
  data: Mode input; PointingE output; SE input; PE input; VE input; NE input; AE input; GE input; ConstraintE output; PointingB output; ConstraintB output
function [PointingE, ConstraintE, PointingB, ConstraintB] = Guidance(Mode,SE,PE,VE,NE,AE,GE)

switch Mode
    case 1%Sun  
        PointingE = SE;
        ConstraintE = VE;
        if dot(SE,cross(VE,PE))>0 %if the sun is on the antinormal side
            PointingB = [1;-1;0];%points the sun negative y
        else %if the sun is on the normal side
            PointingB = [-1;-1;0];%points the sun positive y
        end
        ConstraintB = [0;0;1];
    case 2 %Ground
        PointingE = PE;
        ConstraintE = VE;
        PointingB = [0;0;1];
        ConstraintB = [0;1;0];
    case 3 %Imaging Argentina
        PointingE = AE-PE;
        ConstraintE = VE;
        PointingB = [0;1;0];
        ConstraintB = [0;0;1];
    case 4 %Imaging Namibia
        PointingE = VE;
        ConstraintE = NE-PE;
        PointingB = [0;0;1];
        ConstraintB = [0;1;0];    
    otherwise %Nadir
        PointingE = VE;
        ConstraintE = PE;
        PointingB = [0;0;1];
        ConstraintB = [0;-1;0];
  
end

== matlab function FCS/Guidance/Eclipse Prediction ==
  data: s input; Eclipse output; p input
function Eclipse = fcn(s,p)

if dot(s,p)/(norm(s)*norm(p))<-0.32556815 %angle greater than 109degrees
    Eclipse = 1;
else
    Eclipse = 0 ;
end
